simulink subsystem "PvtSubSys_VSM_ACC_DHT"  (R2020b)
settings: Solver=VariableStepAuto  StartTime=0.0  StopTime=10.0  RelTol=1e-3
values from neighbouring files (symbols this model uses):
  P_VSM_ACC_AutoGoSW = 1.0    [ACC.sldd]
  P_VSM_ACC_BOMEntry_ACCDecReqValue = -0.5    [ACC.sldd]
  P_VSM_ACC_BOMEntry_AxvRefMs2 = -0.5    [ACC.sldd]
  P_VSM_ACC_BOMExit_ACCDecReqValue = -0.3    [ACC.sldd]
  P_VSM_ACC_BrakeOnlyNum = 500.0    [ACC.sldd]
  P_VSM_ACC_RadarOffset = 0.5    [ACC.sldd]
  P_VSM_ACC_StandActiveNumACCMode = 1500.0    [ACC.sldd]
  P_VSM_ACC_StandActiveNumHWAMode = 1500.0    [ACC.sldd]
  P_VSM_ACCExit_AccOverride = 900.0    [ACC.sldd]
  P_VSM_ACCExit_StandWaitTime = 180.0    [ACC.sldd]
  P_VSM_TJA_ActiveWaitNum = 3000.0    [ACC.sldd]
undefined symbols (not defined in the file or in its folder): ACC_STATE, HWAError_Error, HWAError_ErrorBlindness, HWAError_ErrorFast, HWAError_Inhibit, TJA_STATE
libraries: simulink x130, TrueDurationTime x16
(part 2 of 2)

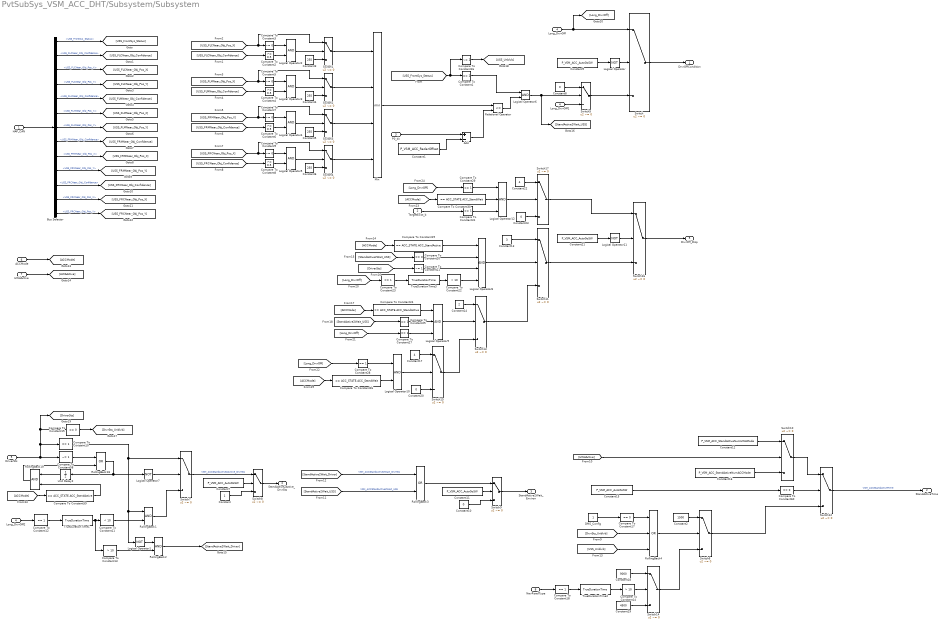
== system PvtSubSys_VSM_ACC_DHT/Subsystem/Subsystem ==
  HAP_CAN : Inport  OutDataTypeStr=Bus: HAP_CAN
  TargetExist_b : Inport  Port=2
  P0_dx : Inport  Port=3
  Long_DrvrOff : Inport  Port=4
  DriverSts : Inport  Port=5
  ACCMode : Inport  Port=6
  HWAActive : Inport  Port=7
  NavRoadType : Inport  Port=8
  Add : Sum  Inputs=+-
  Bus Selector : BusSelector  OutputSignals=USS_FrontSys_Status,USS_FLCNear_Obj_Confidence,USS_FLCNear_Obj_Pos_X,USS_FLCNear_Obj_Pos_Y,USS_FLMNear_Obj_Confidence,USS_FLMNear_Obj_Pos_X,USS_FLMNear_Obj_Pos_Y,USS_FRMNear_Obj_Confidence,USS_FRMNear_Obj_Pos_X,USS_FRMNear_Obj_Pos_Y,USS_FRCNear_Obj_Confidence,USS_FRCNear_Obj_Pos_X,USS_FRCNear_Obj_Pos_Y
  Compare To Constant1 : simulink/Logic and Bit Operations/Compare To Constant  relop===  const=2  OutDataTypeStr=boolean
  Compare To Constant16 : simulink/Logic and Bit Operations/Compare To Constant  relop=~=  const=2  OutDataTypeStr=boolean
  Compare To Constant{2,4,6,8} (4 alike) : simulink/Logic and Bit Operations/Compare To Constant  relop=>=  const=0.5  OutDataTypeStr=boolean
  Compare To Constant{15,17,20,60} (4 alike) : simulink/Logic and Bit Operations/Compare To Constant  relop===  const=0  OutDataTypeStr=boolean
  Compare To Constant21 : simulink/Logic and Bit Operations/Compare To Constant  relop=~=  const=1  OutDataTypeStr=boolean
  Compare To Constant{10,12,18,23,25,27..29,31} (9 alike) : simulink/Logic and Bit Operations/Compare To Constant  relop===  const=1  OutDataTypeStr=boolean
  Compare To Constant{3,5,7,9} (4 alike) : simulink/Logic and Bit Operations/Compare To Constant  relop=~=  const=0  OutDataTypeStr=boolean
  Compare To Constant11 : simulink/Logic and Bit Operations/Compare To Constant  relop=<  const=10  OutDataTypeStr=boolean
  Compare To Constant13 : simulink/Logic and Bit Operations/Compare To Constant  relop=>  const=10  OutDataTypeStr=boolean
  Compare To Constant14 : simulink/Logic and Bit Operations/Compare To Constant  relop=>  const=10  OutDataTypeStr=boolean
  Compare To Constant19 : simulink/Logic and Bit Operations/Compare To Constant  relop===  const=ACC_STATE.ACC_StandActive  OutDataTypeStr=boolean
  Compare To Constant22 : simulink/Logic and Bit Operations/Compare To Constant  relop=<  const=10  OutDataTypeStr=boolean
  Compare To Constant24 : simulink/Logic and Bit Operations/Compare To Constant  relop===  const=ACC_STATE.ACC_StandActive  OutDataTypeStr=boolean
  Compare To Constant26 : simulink/Logic and Bit Operations/Compare To Constant  relop===  const=ACC_STATE.ACC_StandWait  OutDataTypeStr=boolean
  Compare To Constant30 : simulink/Logic and Bit Operations/Compare To Constant  relop===  const=ACC_STATE.ACC_StandWait  OutDataTypeStr=boolean
  Compare To Constant58 : simulink/Logic and Bit Operations/Compare To Constant  relop=~=  const=1  OutDataTypeStr=boolean
  Compare To Constant59 : simulink/Logic and Bit Operations/Compare To Constant  relop===  const=ACC_STATE.ACC_StandActive  OutDataTypeStr=boolean
  Constant : Constant  OutDataTypeStr=boolean
  Constant1 : Constant  Value=P_VSM_ACC_RadarOffset
  Constant10 : Constant  Value=0  OutDataTypeStr=boolean
  Constant{7,9,11,15,21} (5 alike) : Constant  Value=P_VSM_ACC_AutoGoSW  VectorParams1D=off  SampleTime=-1
  Constant12 : Constant  Value=P_VSM_ACC_StandActiveNumHWAMode  VectorParams1D=off  SampleTime=-1
  Constant13 : Constant  Value=3  OutDataTypeStr=uint8
  Constant14 : Constant  Value=2  OutDataTypeStr=uint8
  Constant16 : Constant  Value=P_VSM_ACC_StandActiveNumACCMode  VectorParams1D=off  SampleTime=-1
  Constant17 : Constant  Value=4  OutDataTypeStr=uint8
  Constant18 : Constant  Value=9000  VectorParams1D=off  OutDataTypeStr=uint16  SampleTime=-1
  Constant19 : Constant  Value=4500  VectorParams1D=off  OutDataTypeStr=uint16  SampleTime=-1
  Constant2 : Constant  Value=1500  VectorParams1D=off  OutDataTypeStr=uint16  SampleTime=-1
  Constant20 : Constant  Value=0  OutDataTypeStr=uint8
  Constant22 : Constant  Value=4  OutDataTypeStr=uint8
  Constant23 : Constant  Value=0  OutDataTypeStr=uint8
  Constant{3..6} (4 alike) : Constant  Value=255  OutDataTypeStr=single
  Constant8 : Constant  Value=0  OutDataTypeStr=boolean
  DMS_Config : Constant  OutDataTypeStr=boolean
  Logical Operator{,1,7,11} (4 alike) : Logic  Operator=NOT  Inputs=1  AllPortsSameDT=off  OutDataTypeStr=boolean
  Logical Operator{2..6,10} (6 alike) : Logic  AllPortsSameDT=off  OutDataTypeStr=boolean
  Logical Operator12 : Logic  Inputs=3  AllPortsSameDT=off  OutDataTypeStr=boolean
  Logical Operator8 : Logic  Inputs=4  AllPortsSameDT=off  OutDataTypeStr=boolean
  Logical Operator9 : Logic  Inputs=3  AllPortsSameDT=off  OutDataTypeStr=boolean
  Long_DrvrOff1 : InportShadow  Port=4
  Long_DrvrOff2 : InportShadow  Port=4
  Min : MinMax  Inputs=4
  Relational Operator : RelationalOperator  Operator=<=  OutDataTypeStr=boolean  RndMeth=Simplest
  RollingBack1 : Logic  AllPortsSameDT=off  OutDataTypeStr=boolean
  RollingBack18 : Logic  Operator=OR  AllPortsSameDT=off  OutDataTypeStr=boolean
  RollingBack19 : Logic  AllPortsSameDT=off  OutDataTypeStr=boolean
  RollingBack2 : Logic  AllPortsSameDT=off  OutDataTypeStr=boolean
  RollingBack3 : Logic  Operator=OR  AllPortsSameDT=off  OutDataTypeStr=boolean
  RollingBack4 : Logic  Operator=OR  Inputs=3  AllPortsSameDT=off  OutDataTypeStr=boolean
  Switch{,1..17} (18 alike) : Switch  Criteria=u2 ~= 0
  TrueDurationTime1 : TrueDurationTime/TrueDurationTime  TCycle=0.02
  TrueDurationTime2 : TrueDurationTime/TrueDurationTime  TCycle=0.02
  TrueDurationTime3 : TrueDurationTime/TrueDurationTime  TCycle=0.02
  Unit Delay2 : UnitDelay  SampleTime=-1  HasFrameUpgradeWarning=on
  DrvrOffCondition : Outport
  StandActiveTime : Outport  Port=2
  StandActive2Wait_Environ : Outport  Port=3
  StandActive2Active_DrvrSts : Outport  Port=4
  DrvrOff_Disp : Outport  Port=5
  wires:
  Switch/1 -> DrvrOffCondition/1
  Long_DrvrOff/1 -> [Long_DrvrOff], Switch/1
  Constant9/1 -> Logical Operator/1
  Logical Operator/1 -> Switch/2
  [USS_FrontSys_Status] -> Compare To Constant16/1, Compare To Constant1/1
  [USS_FLCNear_Obj_Confidence] -> Compare To Constant2/1
  Logical Operator2/1 -> Switch1/2
  Compare To Constant2/1 -> Logical Operator2/2
  [USS_FLCNear_Obj_Pos_X] -> Switch1/1, Compare To Constant3/1
  Compare To Constant3/1 -> Logical Operator2/1
  Constant3/1 -> Switch1/3
  Constant4/1 -> Switch2/3
  Compare To Constant5/1 -> Logical Operator3/1
  [USS_FLMNear_Obj_Pos_X] -> Compare To Constant5/1, Switch2/1
  Compare To Constant4/1 -> Logical Operator3/2
  Logical Operator3/1 -> Switch2/2
  [USS_FLMNear_Obj_Confidence] -> Compare To Constant4/1
  [USS_FRMNear_Obj_Confidence] -> Compare To Constant6/1
  Logical Operator4/1 -> Switch3/2
  Compare To Constant6/1 -> Logical Operator4/2
  [USS_FRMNear_Obj_Pos_X] -> Switch3/1, Compare To Constant7/1
  Compare To Constant7/1 -> Logical Operator4/1
  Constant5/1 -> Switch3/3
  Constant6/1 -> Switch4/3
  Compare To Constant9/1 -> Logical Operator5/1
  [USS_FRCNear_Obj_Pos_X] -> Compare To Constant9/1, Switch4/1
  Compare To Constant8/1 -> Logical Operator5/2
  Logical Operator5/1 -> Switch4/2
  [USS_FRCNear_Obj_Confidence] -> Compare To Constant8/1
  Switch2/1 -> Min/2
  Switch1/1 -> Min/1
  Switch3/1 -> Min/3
  Switch4/1 -> Min/4
  Min/1 -> Relational Operator/1
  P0_dx/1 -> Add/1
  Add/1 -> Relational Operator/2
  Constant1/1 -> Add/2
  Compare To Constant1/1 -> Logical Operator6/1
  Relational Operator/1 -> Logical Operator6/2
  Logical Operator6/1 -> [StandActive2Wait_USS], Switch5/2
  Constant8/1 -> Switch5/1
  Long_DrvrOff1/1 -> Switch5/3
  Switch5/1 -> Switch/3
  HAP_CAN/1 -> Bus Selector/1
  Bus Selector/3 -> [USS_FLCNear_Obj_Pos_X]  "<USS_FLCNear_Obj_Pos_X>"
  Bus Selector/2 -> [USS_FLCNear_Obj_Confidence]  "<USS_FLCNear_Obj_Confidence>"
  Bus Selector/4 -> [USS_FLCNear_Obj_Pos_Y]  "<USS_FLCNear_Obj_Pos_Y>"
  Bus Selector/1 -> [USS_FrontSys_Status]  "<USS_FrontSys_Status>"
  Bus Selector/7 -> [USS_FLMNear_Obj_Pos_Y]  "<USS_FLMNear_Obj_Pos_Y>"
  Bus Selector/6 -> [USS_FLMNear_Obj_Pos_X]  "<USS_FLMNear_Obj_Pos_X>"
  Bus Selector/5 -> [USS_FLMNear_Obj_Confidence]  "<USS_FLMNear_Obj_Confidence>"
  Bus Selector/10 -> [USS_FRMNear_Obj_Pos_Y]  "<USS_FRMNear_Obj_Pos_Y>"
  Bus Selector/9 -> [USS_FRMNear_Obj_Pos_X]  "<USS_FRMNear_Obj_Pos_X>"
  Bus Selector/8 -> [USS_FRMNear_Obj_Confidence]  "<USS_FRMNear_Obj_Confidence>"
  Bus Selector/11 -> [USS_FRCNear_Obj_Confidence]  "<USS_FRCNear_Obj_Confidence>"
  Bus Selector/12 -> [USS_FRCNear_Obj_Pos_X]  "<USS_FRCNear_Obj_Pos_X>"
  Bus Selector/13 -> [USS_FRCNear_Obj_Pos_Y]  "<USS_FRCNear_Obj_Pos_Y>"
  Logical Operator7/1 -> Switch7/2
  Compare To Constant58/1 -> RollingBack18/1
  Switch12/1 -> StandActiveTime/1  "VSM_ACCStandActiveTime"
  [ACCMode] -> Compare To Constant59/1
  RollingBack18/1 -> Unit Delay2/1, Logical Operator7/1
  Compare To Constant59/1 -> RollingBack19/2
  Unit Delay2/1 -> RollingBack19/1
  RollingBack19/1 -> RollingBack18/2
  ACCMode/1 -> [ACCMode]
  HWAActive/1 -> [HWAActive]
  DriverSts/1 -> Compare To Constant10/1, Compare To Constant15/1, [DriverSts], Compare To Constant58/1
  Compare To Constant10/1 -> Logical Operator1/1, RollingBack1/1, Switch7/1
  RollingBack1/1 -> Switch7/3
  TrueDurationTime1/1 -> Compare To Constant13/1, Compare To Constant11/1
  Compare To Constant11/1 -> RollingBack1/2
  Long_DrvrOff2/1 -> Compare To Constant12/1
  Compare To Constant12/1 -> TrueDurationTime1/1
  Logical Operator1/1 -> RollingBack2/1
  Compare To Constant13/1 -> RollingBack2/2
  RollingBack2/1 -> [StandActive2Wait_Driver]
  [StandActive2Wait_Driver] -> RollingBack3/1  "VSM_ACCStandActive2Wait_DrvrSts"
  [StandActive2Wait_USS] -> RollingBack3/2  "VSM_ACCStandActive2Wait_USS"
  RollingBack3/1 -> Switch9/1
  Switch7/1 -> Switch8/1  "VSM_ACCStandActive2Active_DrvrSts"
  Switch8/1 -> StandActive2Active_DrvrSts/1
  Constant7/1 -> Switch8/2
  Constant/1 -> Switch8/3
  Constant10/1 -> Switch9/3
  Constant11/1 -> Switch9/2
  Switch9/1 -> StandActive2Wait_Environ/1
  [HWAActive] -> Switch10/2
  Constant12/1 -> Switch10/1
  Switch6/1 -> Switch12/3
  Switch10/1 -> Switch12/1
  Constant15/1 -> Compare To Constant60/1
  Compare To Constant60/1 -> Switch12/2
  Constant16/1 -> Switch10/3
  Compare To Constant15/1 -> [DrvrSts_Unblvb]
  Compare To Constant16/1 -> [USS_Unblvb]
  DMS_Config/1 -> Compare To Constant17/1
  Compare To Constant17/1 -> RollingBack4/1
  [DrvrSts_Unblvb] -> RollingBack4/2
  [USS_Unblvb] -> RollingBack4/3
  RollingBack4/1 -> Switch6/2
  Constant2/1 -> Switch6/1
  Switch14/1 -> Switch6/3
  NavRoadType/1 -> Compare To Constant18/1
  Compare To Constant18/1 -> TrueDurationTime2/1
  Constant18/1 -> Switch14/1
  Constant19/1 -> Switch14/3
  TrueDurationTime2/1 -> Compare To Constant14/1
  Compare To Constant14/1 -> Switch14/2
  [ACCMode] -> Compare To Constant19/1
  Logical Operator8/1 -> Switch11/2
  Compare To Constant19/1 -> Logical Operator8/1
  [StandActive2Wait_USS] -> Compare To Constant20/1
  Compare To Constant20/1 -> Logical Operator8/2
  Compare To Constant21/1 -> Logical Operator8/3
  [DriverSts] -> Compare To Constant21/1
  Compare To Constant23/1 -> TrueDurationTime3/1
  TrueDurationTime3/1 -> Compare To Constant22/1
  [Long_DrvrOff] -> Compare To Constant23/1
  Compare To Constant22/1 -> Logical Operator8/4
  Constant13/1 -> Switch11/1
  Switch13/1 -> Switch11/3
  Logical Operator9/1 -> Switch13/2
  [ACCMode] -> Compare To Constant24/1
  Compare To Constant24/1 -> Logical Operator9/1
  [StandActive2Wait_USS] -> Compare To Constant25/1
  Compare To Constant25/1 -> Logical Operator9/2
  Constant14/1 -> Switch13/1
  [ACCMode] -> Compare To Constant26/1
  Switch15/1 -> Switch13/3
  Logical Operator10/1 -> Switch15/2
  Compare To Constant26/1 -> Logical Operator10/2
  [Long_DrvrOff] -> Compare To Constant27/1
  Compare To Constant27/1 -> Logical Operator9/3
  Compare To Constant28/1 -> Logical Operator10/1
  [Long_DrvrOff] -> Compare To Constant28/1
  Constant17/1 -> Switch15/1
  Constant20/1 -> Switch15/3
  Logical Operator11/1 -> Switch16/2
  Constant21/1 -> Logical Operator11/1
  Switch11/1 -> Switch16/3
  Constant23/1 -> Switch17/3
  Constant22/1 -> Switch17/1
  [Long_DrvrOff] -> Compare To Constant29/1
  Compare To Constant29/1 -> Logical Operator12/1
  Compare To Constant30/1 -> Logical Operator12/2
  Logical Operator12/1 -> Switch17/2
  [ACCMode] -> Compare To Constant30/1
  Switch17/1 -> Switch16/1
  TargetExist_b/1 -> Compare To Constant31/1
  Compare To Constant31/1 -> Logical Operator12/3
  Switch16/1 -> DrvrOff_Disp/1

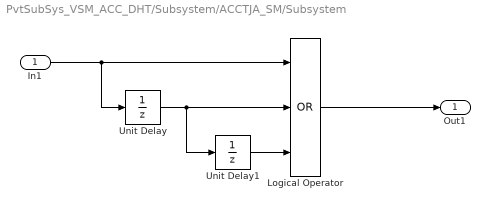
== system PvtSubSys_VSM_ACC_DHT/Subsystem/ACCTJA_SM/Subsystem ==
  In1 : Inport
  Logical Operator : Logic  Operator=OR  Inputs=3  AllPortsSameDT=off  OutDataTypeStr=boolean
  Unit Delay : UnitDelay  SampleTime=-1  HasFrameUpgradeWarning=on
  Unit Delay1 : UnitDelay  SampleTime=-1  HasFrameUpgradeWarning=on
  Out1 : Outport
  wires:
  In1/1 -> Logical Operator/1, Unit Delay/1
  Unit Delay/1 -> Logical Operator/2, Unit Delay1/1
  Logical Operator/1 -> Out1/1
  Unit Delay1/1 -> Logical Operator/3

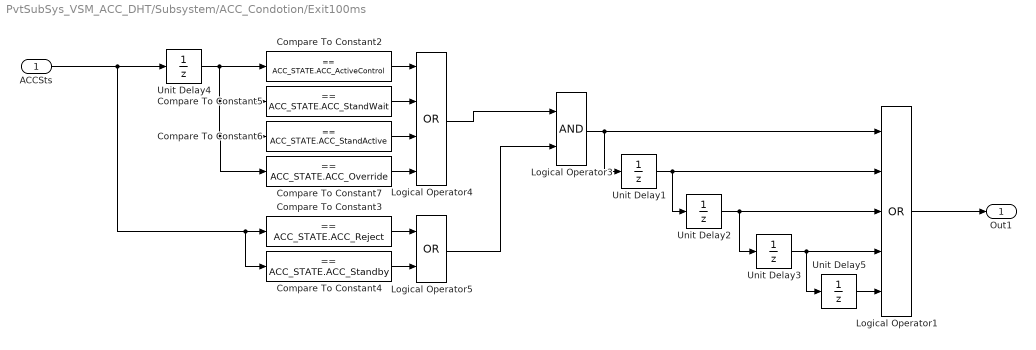
== system PvtSubSys_VSM_ACC_DHT/Subsystem/ACC_Condotion/Exit100ms ==
  ACCSts : Inport
  Compare To Constant2 : simulink/Logic and Bit Operations/Compare To Constant  relop===  const=ACC_STATE.ACC_ActiveControl  OutDataTypeStr=boolean
  Compare To Constant3 : simulink/Logic and Bit Operations/Compare To Constant  relop===  const=ACC_STATE.ACC_Reject  OutDataTypeStr=boolean
  Compare To Constant4 : simulink/Logic and Bit Operations/Compare To Constant  relop===  const=ACC_STATE.ACC_Standby  OutDataTypeStr=boolean
  Compare To Constant5 : simulink/Logic and Bit Operations/Compare To Constant  relop===  const=ACC_STATE.ACC_StandWait  OutDataTypeStr=boolean
  Compare To Constant6 : simulink/Logic and Bit Operations/Compare To Constant  relop===  const=ACC_STATE.ACC_StandActive  OutDataTypeStr=boolean
  Compare To Constant7 : simulink/Logic and Bit Operations/Compare To Constant  relop===  const=ACC_STATE.ACC_Override  OutDataTypeStr=boolean
  Logical Operator1 : Logic  Operator=OR  Inputs=5  AllPortsSameDT=off  OutDataTypeStr=boolean
  Logical Operator3 : Logic  AllPortsSameDT=off  OutDataTypeStr=boolean
  Logical Operator4 : Logic  Operator=OR  Inputs=4  AllPortsSameDT=off  OutDataTypeStr=boolean
  Logical Operator5 : Logic  Operator=OR  AllPortsSameDT=off  OutDataTypeStr=boolean
  Unit Delay{1..3,5} (4 alike) : UnitDelay  SampleTime=-1  HasFrameUpgradeWarning=on
  Unit Delay4 : UnitDelay  InitialCondition=ACC_STATE.ACC_Off  SampleTime=-1  HasFrameUpgradeWarning=on
  Out1 : Outport
  wires:
  Unit Delay5/1 -> Logical Operator1/5
  Unit Delay3/1 -> Logical Operator1/4, Unit Delay5/1
  Unit Delay2/1 -> Logical Operator1/3, Unit Delay3/1
  Unit Delay1/1 -> Logical Operator1/2, Unit Delay2/1
  Logical Operator3/1 -> Unit Delay1/1, Logical Operator1/1
  Compare To Constant7/1 -> Logical Operator4/4
  Compare To Constant6/1 -> Logical Operator4/3
  Compare To Constant5/1 -> Logical Operator4/2
  Compare To Constant2/1 -> Logical Operator4/1
  Compare To Constant3/1 -> Logical Operator5/1
  Compare To Constant4/1 -> Logical Operator5/2
  ACCSts/1 -> Compare To Constant4/1, Compare To Constant3/1, Unit Delay4/1
  Unit Delay4/1 -> Compare To Constant5/1, Compare To Constant6/1, Compare To Constant7/1, Compare To Constant2/1
  Logical Operator4/1 -> Logical Operator3/1
  Logical Operator1/1 -> Out1/1
  Logical Operator5/1 -> Logical Operator3/2

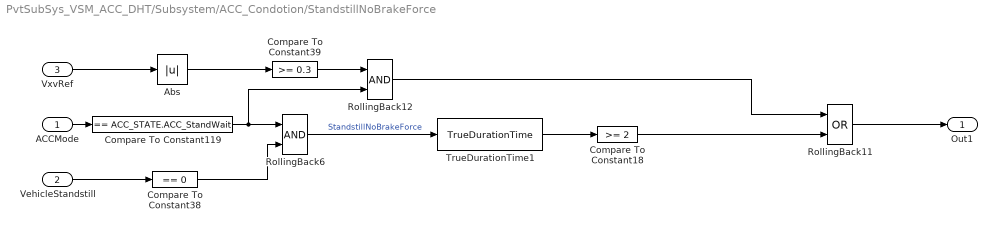
== system PvtSubSys_VSM_ACC_DHT/Subsystem/ACC_Condotion/StandstillNoBrakeForce ==
  ACCMode : Inport
  VehicleStandstill : Inport  Port=2
  VxvRef : Inport  Port=3
  Abs : Abs
  Compare To Constant119 : simulink/Logic and Bit Operations/Compare To Constant  relop===  const=ACC_STATE.ACC_StandWait  OutDataTypeStr=boolean
  Compare To Constant18 : simulink/Logic and Bit Operations/Compare To Constant  relop=>=  const=2  OutDataTypeStr=boolean
  Compare To Constant38 : simulink/Logic and Bit Operations/Compare To Constant  relop===  const=0  OutDataTypeStr=boolean
  Compare To Constant39 : simulink/Logic and Bit Operations/Compare To Constant  relop=>=  const=0.3  OutDataTypeStr=boolean
  RollingBack11 : Logic  Operator=OR  AllPortsSameDT=off  OutDataTypeStr=boolean
  RollingBack12 : Logic  AllPortsSameDT=off  OutDataTypeStr=boolean
  RollingBack6 : Logic  AllPortsSameDT=off  OutDataTypeStr=boolean
  TrueDurationTime1 : TrueDurationTime/TrueDurationTime  TCycle=0.02
  Out1 : Outport
  wires:
  Abs/1 -> Compare To Constant39/1
  Compare To Constant119/1 -> RollingBack6/1, RollingBack12/2
  RollingBack6/1 -> TrueDurationTime1/1  "StandstillNoBrakeForce"
  TrueDurationTime1/1 -> Compare To Constant18/1
  Compare To Constant38/1 -> RollingBack6/2
  VehicleStandstill/1 -> Compare To Constant38/1
  Compare To Constant39/1 -> RollingBack12/1
  RollingBack12/1 -> RollingBack11/1
  RollingBack11/1 -> Out1/1
  VxvRef/1 -> Abs/1
  Compare To Constant18/1 -> RollingBack11/2
  ACCMode/1 -> Compare To Constant119/1

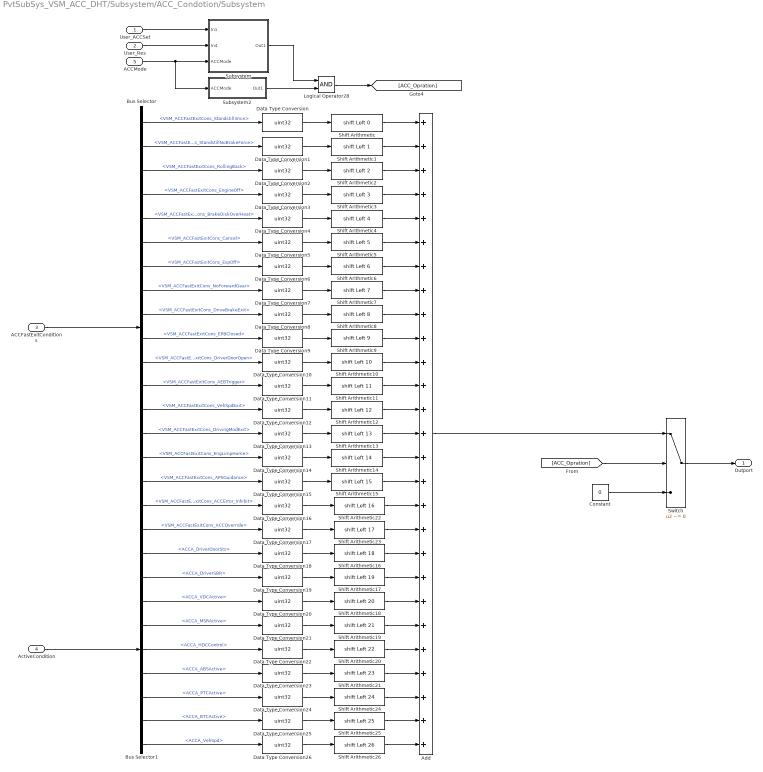
== system PvtSubSys_VSM_ACC_DHT/Subsystem/ACC_Condotion/Subsystem ==
  User_ACCSet : Inport
  User_Res : Inport  Port=2
  ACCFastExitConditions : Inport  Port=3
  ActiveCondition : Inport  Port=4
  ACCMode : Inport  Port=5
  Add : Sum  Inputs=+++++++++++++++++++++++++++
  Bus Selector : BusSelector  OutputSignals=VSM_ACCFastExitCons_Standstill3min,VSM_ACCFastExitCons_StandstillNoBrakeForce,VSM_ACCFastExitCons_RollingBack,VSM_ACCFastExitCons_EngineOff,VSM_ACCFastExitCons_BrakeDiskOverHeat,VSM_ACCFastExitCons_Cancel,VSM_ACCFastExitCons_EspOff,VSM_ACCFastExitCons_NoForwardGear,VSM_ACCFastExitCons_DriveBrakeExit,VSM_ACCFastExitCons_EPBClosed,VSM_ACCFastExitCons_DriverDoorOpen,VSM_ACCFastExitCons_AEBTrigger,VSM_ACCFastExitCons_VehSpdExit,VSM_ACCFastExitCons_DrivingModExit,VSM_ACCFastExitCons_EngLimpHome,VSM_ACCFastExitCons_APSGuidance,VSM_ACCFastExitCons_ACCError_Inhibit,VSM_ACCFastExitCons_ACCOverride
  Bus Selector1 : BusSelector  OutputSignals=ACCA_DriverDoorSts,ACCA_DriverSBR,ACCA_VDCActive,ACCA_MSRActive,ACCA_HDCControl,ACCA_ABSActive,ACCA_PTCActive,ACCA_BTCActive,ACCA_VehSpd
  Constant : Constant  Value=0  OutDataTypeStr=uint32
  Data Type Conversion{,1..26} (27 alike) : DataTypeConversion  OutDataTypeStr=uint32
  Logical Operator28 : Logic  AllPortsSameDT=off  OutDataTypeStr=boolean
  Shift Arithmetic : ArithShift  BitShiftDirection=Left
  Shift Arithmetic1 : ArithShift  BitShiftNumber=1  BitShiftDirection=Left
  Shift Arithmetic10 : ArithShift  BitShiftNumber=10  BitShiftDirection=Left
  Shift Arithmetic11 : ArithShift  BitShiftNumber=11  BitShiftDirection=Left
  Shift Arithmetic12 : ArithShift  BitShiftNumber=12  BitShiftDirection=Left
  Shift Arithmetic13 : ArithShift  BitShiftNumber=13  BitShiftDirection=Left
  Shift Arithmetic14 : ArithShift  BitShiftNumber=14  BitShiftDirection=Left
  Shift Arithmetic15 : ArithShift  BitShiftNumber=15  BitShiftDirection=Left
  Shift Arithmetic16 : ArithShift  BitShiftNumber=18  BitShiftDirection=Left
  Shift Arithmetic17 : ArithShift  BitShiftNumber=19  BitShiftDirection=Left
  Shift Arithmetic18 : ArithShift  BitShiftNumber=20  BitShiftDirection=Left
  Shift Arithmetic19 : ArithShift  BitShiftNumber=21  BitShiftDirection=Left
  Shift Arithmetic2 : ArithShift  BitShiftNumber=2  BitShiftDirection=Left
  Shift Arithmetic20 : ArithShift  BitShiftNumber=22  BitShiftDirection=Left
  Shift Arithmetic21 : ArithShift  BitShiftNumber=23  BitShiftDirection=Left
  Shift Arithmetic22 : ArithShift  BitShiftNumber=16  BitShiftDirection=Left
  Shift Arithmetic23 : ArithShift  BitShiftNumber=17  BitShiftDirection=Left
  Shift Arithmetic24 : ArithShift  BitShiftNumber=24  BitShiftDirection=Left
  Shift Arithmetic25 : ArithShift  BitShiftNumber=25  BitShiftDirection=Left
  Shift Arithmetic26 : ArithShift  BitShiftNumber=26  BitShiftDirection=Left
  Shift Arithmetic3 : ArithShift  BitShiftNumber=3  BitShiftDirection=Left
  Shift Arithmetic4 : ArithShift  BitShiftNumber=4  BitShiftDirection=Left
  Shift Arithmetic5 : ArithShift  BitShiftNumber=5  BitShiftDirection=Left
  Shift Arithmetic6 : ArithShift  BitShiftNumber=6  BitShiftDirection=Left
  Shift Arithmetic7 : ArithShift  BitShiftNumber=7  BitShiftDirection=Left
  Shift Arithmetic8 : ArithShift  BitShiftNumber=8  BitShiftDirection=Left
  Shift Arithmetic9 : ArithShift  BitShiftNumber=9  BitShiftDirection=Left
  Subsystem : Subsystem
  Subsystem2 : Subsystem
  Switch : Switch  Criteria=u2 ~= 0
  Outport : Outport
  wires:
  Switch/1 -> Outport/1
  [ACC_Opration] -> Switch/2
  Logical Operator28/1 -> [ACC_Opration]
  Subsystem2/1(Out1) -> Logical Operator28/2
  Subsystem/1(Out1) -> Logical Operator28/1
  User_Res/1 -> Subsystem/2(In4)
  ACCMode/1 -> Subsystem/3(ACCMode), Subsystem2/1(ACCMode)
  User_ACCSet/1 -> Subsystem/1(In1)
  Constant/1 -> Switch/3
  Add/1 -> Switch/1
  Shift Arithmetic15/1 -> Add/16
  Shift Arithmetic14/1 -> Add/15
  Shift Arithmetic13/1 -> Add/14
  Shift Arithmetic12/1 -> Add/13
  Shift Arithmetic11/1 -> Add/12
  Shift Arithmetic10/1 -> Add/11
  Shift Arithmetic9/1 -> Add/10
  Shift Arithmetic8/1 -> Add/9
  Shift Arithmetic7/1 -> Add/8
  Shift Arithmetic6/1 -> Add/7
  Shift Arithmetic5/1 -> Add/6
  Shift Arithmetic4/1 -> Add/5
  Shift Arithmetic3/1 -> Add/4
  Shift Arithmetic2/1 -> Add/3
  Shift Arithmetic1/1 -> Add/2
  Shift Arithmetic/1 -> Add/1
  Shift Arithmetic26/1 -> Add/27
  Shift Arithmetic25/1 -> Add/26
  Shift Arithmetic24/1 -> Add/25
  Shift Arithmetic21/1 -> Add/24
  Shift Arithmetic20/1 -> Add/23
  Shift Arithmetic19/1 -> Add/22
  Shift Arithmetic18/1 -> Add/21
  Shift Arithmetic17/1 -> Add/20
  Shift Arithmetic16/1 -> Add/19
  Shift Arithmetic23/1 -> Add/18
  Shift Arithmetic22/1 -> Add/17
  Data Type Conversion26/1 -> Shift Arithmetic26/1
  Data Type Conversion25/1 -> Shift Arithmetic25/1
  Data Type Conversion24/1 -> Shift Arithmetic24/1
  Data Type Conversion23/1 -> Shift Arithmetic21/1
  Data Type Conversion22/1 -> Shift Arithmetic20/1
  Data Type Conversion21/1 -> Shift Arithmetic19/1
  Data Type Conversion20/1 -> Shift Arithmetic18/1
  Data Type Conversion19/1 -> Shift Arithmetic17/1
  Data Type Conversion18/1 -> Shift Arithmetic16/1
  Data Type Conversion17/1 -> Shift Arithmetic23/1
  Data Type Conversion16/1 -> Shift Arithmetic22/1
  Data Type Conversion15/1 -> Shift Arithmetic15/1
  Data Type Conversion14/1 -> Shift Arithmetic14/1
  Data Type Conversion13/1 -> Shift Arithmetic13/1
  Data Type Conversion12/1 -> Shift Arithmetic12/1
  Data Type Conversion11/1 -> Shift Arithmetic11/1
  Data Type Conversion10/1 -> Shift Arithmetic10/1
  Data Type Conversion9/1 -> Shift Arithmetic9/1
  Data Type Conversion8/1 -> Shift Arithmetic8/1
  Data Type Conversion7/1 -> Shift Arithmetic7/1
  Data Type Conversion6/1 -> Shift Arithmetic6/1
  Data Type Conversion5/1 -> Shift Arithmetic5/1
  Data Type Conversion4/1 -> Shift Arithmetic4/1
  Data Type Conversion3/1 -> Shift Arithmetic3/1
  Data Type Conversion2/1 -> Shift Arithmetic2/1
  Data Type Conversion1/1 -> Shift Arithmetic1/1
  Data Type Conversion/1 -> Shift Arithmetic/1
  Bus Selector1/9 -> Data Type Conversion26/1  "<ACCA_VehSpd>"
  Bus Selector1/8 -> Data Type Conversion25/1  "<ACCA_BTCActive>"
  Bus Selector1/7 -> Data Type Conversion24/1  "<ACCA_PTCActive>"
  Bus Selector1/6 -> Data Type Conversion23/1  "<ACCA_ABSActive>"
  Bus Selector1/5 -> Data Type Conversion22/1  "<ACCA_HDCControl>"
  Bus Selector1/4 -> Data Type Conversion21/1  "<ACCA_MSRActive>"
  Bus Selector1/3 -> Data Type Conversion20/1  "<ACCA_VDCActive>"
  Bus Selector1/1 -> Data Type Conversion18/1  "<ACCA_DriverDoorSts>"
  Bus Selector1/2 -> Data Type Conversion19/1  "<ACCA_DriverSBR>"
  Bus Selector/18 -> Data Type Conversion17/1  "<VSM_ACCFastExitCons_ACCOverride>"
  Bus Selector/17 -> Data Type Conversion16/1  "<VSM_ACCFastExitCons_ACCError_Inhibit>"
  Bus Selector/16 -> Data Type Conversion15/1  "<VSM_ACCFastExitCons_APSGuidance>"
  Bus Selector/15 -> Data Type Conversion14/1  "<VSM_ACCFastExitCons_EngLimpHome>"
  Bus Selector/14 -> Data Type Conversion13/1  "<VSM_ACCFastExitCons_DrivingModExit>"
  Bus Selector/13 -> Data Type Conversion12/1  "<VSM_ACCFastExitCons_VehSpdExit>"
  Bus Selector/12 -> Data Type Conversion11/1  "<VSM_ACCFastExitCons_AEBTrigger>"
  Bus Selector/11 -> Data Type Conversion10/1  "<VSM_ACCFastExitCons_DriverDoorOpen>"
  Bus Selector/10 -> Data Type Conversion9/1  "<VSM_ACCFastExitCons_EPBClosed>"
  Bus Selector/9 -> Data Type Conversion8/1  "<VSM_ACCFastExitCons_DriveBrakeExit>"
  Bus Selector/8 -> Data Type Conversion7/1  "<VSM_ACCFastExitCons_NoForwardGear>"
  Bus Selector/7 -> Data Type Conversion6/1  "<VSM_ACCFastExitCons_EspOff>"
  Bus Selector/6 -> Data Type Conversion5/1  "<VSM_ACCFastExitCons_Cancel>"
  Bus Selector/5 -> Data Type Conversion4/1  "<VSM_ACCFastExitCons_BrakeDiskOverHeat>"
  Bus Selector/4 -> Data Type Conversion3/1  "<VSM_ACCFastExitCons_EngineOff>"
  Bus Selector/3 -> Data Type Conversion2/1  "<VSM_ACCFastExitCons_RollingBack>"
  Bus Selector/2 -> Data Type Conversion1/1  "<VSM_ACCFastExitCons_StandstillNoBrakeForce>"
  Bus Selector/1 -> Data Type Conversion/1  "<VSM_ACCFastExitCons_Standstill3min>"
  ActiveCondition/1 -> Bus Selector1/1
  ACCFastExitConditions/1 -> Bus Selector/1

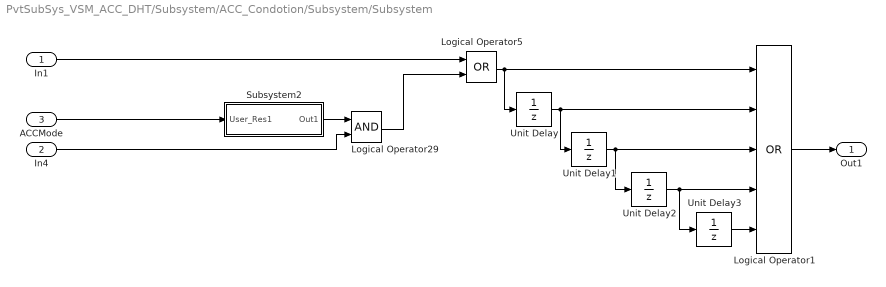
== system PvtSubSys_VSM_ACC_DHT/Subsystem/ACC_Condotion/Subsystem/Subsystem ==
  In1 : Inport
  In4 : Inport  Port=2
  ACCMode : Inport  Port=3
  Logical Operator1 : Logic  Operator=OR  Inputs=5  AllPortsSameDT=off  OutDataTypeStr=boolean
  Logical Operator29 : Logic  AllPortsSameDT=off  OutDataTypeStr=boolean
  Logical Operator5 : Logic  Operator=OR  AllPortsSameDT=off  OutDataTypeStr=boolean
  Subsystem2 : Subsystem
  Unit Delay{,1..3} (4 alike) : UnitDelay  SampleTime=-1  HasFrameUpgradeWarning=on
  Out1 : Outport
  wires:
  Unit Delay3/1 -> Logical Operator1/5
  Unit Delay2/1 -> Logical Operator1/4, Unit Delay3/1
  Unit Delay1/1 -> Logical Operator1/3, Unit Delay2/1
  Logical Operator1/1 -> Out1/1
  Unit Delay/1 -> Logical Operator1/2, Unit Delay1/1
  In1/1 -> Logical Operator5/1
  Logical Operator5/1 -> Unit Delay/1, Logical Operator1/1
  In4/1 -> Logical Operator29/2
  ACCMode/1 -> Subsystem2/1(User_Res1)
  Logical Operator29/1 -> Logical Operator5/2
  Subsystem2/1(Out1) -> Logical Operator29/1

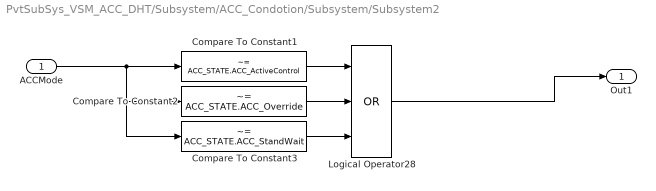
== system PvtSubSys_VSM_ACC_DHT/Subsystem/ACC_Condotion/Subsystem/Subsystem2 ==
  ACCMode : Inport
  Compare To Constant1 : simulink/Logic and Bit Operations/Compare To Constant  relop=~=  const=ACC_STATE.ACC_ActiveControl  OutDataTypeStr=boolean
  Compare To Constant2 : simulink/Logic and Bit Operations/Compare To Constant  relop=~=  const=ACC_STATE.ACC_Override  OutDataTypeStr=boolean
  Compare To Constant3 : simulink/Logic and Bit Operations/Compare To Constant  relop=~=  const=ACC_STATE.ACC_StandWait  OutDataTypeStr=boolean
  Logical Operator28 : Logic  Operator=OR  Inputs=3  AllPortsSameDT=off  OutDataTypeStr=boolean
  Out1 : Outport
  wires:
  Compare To Constant3/1 -> Logical Operator28/3
  Compare To Constant2/1 -> Logical Operator28/2
  Compare To Constant1/1 -> Logical Operator28/1
  ACCMode/1 -> Compare To Constant1/1, Compare To Constant2/1, Compare To Constant3/1
  Logical Operator28/1 -> Out1/1

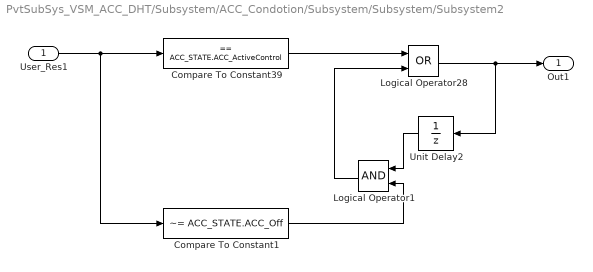
== system PvtSubSys_VSM_ACC_DHT/Subsystem/ACC_Condotion/Subsystem/Subsystem/Subsystem2 ==
  User_Res1 : Inport
  Compare To Constant1 : simulink/Logic and Bit Operations/Compare To Constant  relop=~=  const=ACC_STATE.ACC_Off  OutDataTypeStr=boolean
  Compare To Constant39 : simulink/Logic and Bit Operations/Compare To Constant  relop===  const=ACC_STATE.ACC_ActiveControl  OutDataTypeStr=boolean
  Logical Operator1 : Logic  AllPortsSameDT=off  OutDataTypeStr=boolean
  Logical Operator28 : Logic  Operator=OR  AllPortsSameDT=off  OutDataTypeStr=boolean
  Unit Delay2 : UnitDelay  SampleTime=-1  HasFrameUpgradeWarning=on
  Out1 : Outport
  wires:
  Compare To Constant1/1 -> Logical Operator1/2
  Logical Operator1/1 -> Logical Operator28/2
  User_Res1/1 -> Compare To Constant1/1, Compare To Constant39/1
  Unit Delay2/1 -> Logical Operator1/1
  Logical Operator28/1 -> Unit Delay2/1, Out1/1
  Compare To Constant39/1 -> Logical Operator28/1

== matlab function PvtSubSys_VSM_ACC_DHT/Subsystem/ACC_Condotion/MATLAB Function ==
  data: DriveBrake input; VehicleStandstill input; ActiveConditionsFulfilled output; ActiveEnable input
function ActiveConditionsFulfilled = fcn(DriveBrake,VehicleStandstill,ActiveEnable)
%#codegen
if DriveBrake
    if VehicleStandstill && ActiveEnable
        ActiveConditionsFulfilled = 1;
    else
        ActiveConditionsFulfilled = 0;
    end
else  
    if ActiveEnable
        ActiveConditionsFulfilled = 1;
    else
        ActiveConditionsFulfilled = 0;
    end   
end

== stateflow chart PvtSubSys_VSM_ACC_DHT/Subsystem/ACCTJA_SM/TJA_ACC1 ==
  state ACC_Main [parallel]
    settings: executionOrder=1
    state P
      (history)
      state Off
        entry:
        ACCSts=ACC_Off;
      state Passive
        state Reject
          entry:
          ACCSts=ACC_Reject;
          DriveOffReq=0;
        state Standby
          entry:
          ACCSts=ACC_Standby;
          DriveOffReq=0;
        (default) -> Reject
        Standby -> Reject [order 1] : [ACCActCondF_b==0]//抑制
        Reject -> Standby : [ACCActCondF_b==1]//无抑制
      (default) -> Off
      Off -> Passive : [((ACC_ON==true)||...
          | (TJA_ON==true))&&...
          | (VehConfigACC==1)]
      Passive -> Off : [((ACC_ON==false)&&...
          | (TJA_ON==false))||...
          | (VehConfigACC==0)]
    state Error
      entry:
      ACCSts=ACC_Failure;
    state ACC_Control
      state Brake_Only
        entry:
        BrakeOnlyNum=0;
        ACCSts=ACC_BrakeOnly;
        DriveOffReq=0;
        during:
        BrakeOnlyNum=min(BrakeOnlyNum+1,600);
      state Active
        entry:ActiveNum=1;
        state StandActive
          entry:
          ACCSts=ACC_StandActive;
          StandActiveNum=0;
          DriveOffReq=0;
          during:
          StandActiveNum=min(StandActiveNum+1,20000);
        state StandWait
          entry:
          ACCSts=ACC_StandWait;
          StandWaitNum=0;
          during:
          StandWaitNum=min(StandWaitNum+1,20000);
          exit:
          StandWaitNum=0;
        state ActiveControl
          entry:
          ACCSts=ACC_ActiveControl;
          ActiveControlNum=1;
          during:
          ActiveControlNum=min(ActiveControlNum+1,600);
          DriveOffReq=(DriveOffCondF_b*VehicleStandstill) || (CDDactive*VehicleStandstill*DriveOffReq*(ActiveControlNum<=200));
        state Suspend
          entry:
          ACCSts=ACC_Override;
          AccOverrideNum=0;
          during:
          AccOverrideNum=min(45000,AccOverrideNum+1);
          DriveOffReq=CDDactive*VehicleStandstill*DriveOffReq*(ActiveControlNum<=200);
          exit:
          AccOverrideNum=0;
        StandActive -> Suspend [order 3] : [AccOverride==1]
        (junction 263) -> StandActive [order 2]
        ActiveControl -> StandActive [order 1] : [(VehicleStandstill==1)&&...
            | (DriverBrake==0)&&...
            | (DriveOffCondF_b~=1)]
        StandActive -> ActiveControl [order 1] : [(DriveOffCondF_b==1)&&...
            | (StandActive2Active_DrvrSts==1)&&...
            | (DriverBrake==0)]/DriveOffReq=1;
        StandActive -> StandWait [order 2] : [(VehicleStandstill==1)&&...
            | ((StandActiveNum>...
            | ACC_StandActiveNum)||...
            | (StandActive2Wait_Environ==1))]
        StandWait -> StandActive [order 1] : [(DriverBrake==0)&&...
            | (DriveOffCondF_b==0)&&...
            | ((AccPedalTouch==1)||(Switch_Res==true))]
        StandWait -> Suspend [order 2] : [AccOverride==1]
        StandWait -> ActiveControl [order 3] : [(DriverBrake==0)&&...
            | (DriveOffCondF_b==1)&&...
            | ((AccPedalTouch==1)||...
            | (Switch_Res==true))]...
            | /DriveOffReq=1;
        ActiveControl -> StandWait [order 3] : [(VehicleStandstill==1)&&...
            | (DriverBrake==1)]
        (default) -> (junction 261)
        (junction 261) -> (junction 263) [order 2]
        (junction 263) -> ActiveControl [order 1] : [VehicleStandstill==0]
        (junction 261) -> Suspend [order 1] : [AccOverride==1]
        Suspend -> ActiveControl [order 2] : [AccOverride==0]
        ActiveControl -> Suspend [order 4] : [AccOverride==1]
      ActiveControl -> Brake_Only [order 2] : [(ACCSlowExit_b==1)&&...
          | (ACCDecEnableBOM==1)]
    (default) -> P
    Error -> P : [ACCFailure==0]
    P -> Error : [ACCFailure==1]
    ACC_Control -> Off [order 2] : [(ACC_ON==false)&&...
        | (TJA_ON==false)]
    ACC_Control -> Error [order 1] : [TJAActive~=1&&...
        | ACCFailure==1]
    Suspend -> Passive [order 1] : [ACCSlowExit_b==1]
    Standby -> (junction 259) [order 2] : [(ACC_ON==true)&&...
        | (Switch_Set==true)]
    Standby -> (junction 259) [order 3] : [(ACC_ON==true)&&...
        | (Switch_Res==true)&&...//Res了
        | (ActiveNum>0)]//ActiveNum用以区分激活还是复位
    Brake_Only -> Passive : [(BrakeOnlyNum>P_VSM_ACC_BrakeOnlyNum)||...//breakonly超过10s
        | (ACCDecDisableBOM==1)||...
        | (AccOverride==1)||...
        | (VehicleStandstill==1)||...//车辆静止
        | (NoTarget==1)||...//无目标
        | (ACCFastExit_b==1)]
    Active -> Passive : [(ACCFastExit_b==1)||...
        | ((ACCSlowExit_b==1)&&...
        | (ACCDecEnableBOM~=1))]
    (junction 259) -> Active
  data: StandActiveNum local uint16; ACC_ON input boolean size=1; TJA_ON input boolean size=1; CDDactive input size=1; VehicleStandstill input size=1; ACCFailure input size=1; ACCActCondF_b input size=1; DriveOffCondF_b input size=1; AccOverride input size=1; ActiveNum local uint16 size=1 [0..100] =0; ACCFastExit_b input size=1; ACCSlowExit_b input size=1; StandWaitNum output uint16 size=1 =0; ActiveControlNum local uint16 size=1 =0; BrakeOnlyNum local uint16 size=1 =0; DriverBrake input size=1; DriveOffReq output boolean size=1 =0; NoTarget input size=1; AccPedalTouch input size=1; ACCSts output Enum: ACC_STATE size=1 =ACC_STATE.ACC_Off; Switch_Set input boolean size=1 =false; Switch_Res input boolean size=1 =false; VehConfigTJA input boolean; VehConfigACC input boolean; ACCDecEnableBOM input boolean size=1; ACCDecDisableBOM input boolean size=1; ActiveWaitNum local uint16 size=1; AccOverrideNum local uint16 size=1 [0..100] =0; P_VSM_ACC_BrakeOnlyNum parameter uint16; ACC_StandActiveNum input; StandActive2Wait_Environ input; StandActive2Active_DrvrSts input; cnt local uint16; SafeStopNum local uint16; TJAActive input boolean

== stateflow chart PvtSubSys_VSM_ACC_DHT/Subsystem/ACCTJA_SM/TJA_ACC2 ==
  state TJA_Main [parallel]
    settings: executionOrder=1
    state Off
      en:
      TJASts=TJA_Off;
    state TJAOn
      state Error
        en:
        TJASts=TJA_Error;
      state W
        state Ready
          en:
          TJASts=TJA_Ready;
        state Idle
          en:
          TJASts=TJA_Idle;
        state Active
          en:
          TJASts=TJA_Active;
          cnt=0;
          du:
          cnt=min(10,cnt+1)
        state Wait
          en:
          TJASts=TJA_Wait;
          du:
          ActiveWaitNum=min(3000,ActiveWaitNum+1);
          ex:
          ActiveWaitNum=0;
        state Idle1
          en:
          TJASts=TJA_Idle;
          TJASafeStopExit_b=false;
        state Recover
          en:
          TJASts=TJA_Ready;
        state SafeStop
          en:
          TJASts=TJA_SafeStop;
          du:
          SafeStopNum=min(300,SafeStopNum+1);
          TJASafeStopExit_b=(SafeStopNum>250);
          ACCParkShiftReq_b=VehicleStandstill;
          ex:
          TJAStopExit=true;
          ACCParkShiftReq_b=false;
          SafeStopNum=0;
        (junction 438) -> Idle [order 1] : [(ACCSts==ACC_Reject)||...
            | (TJA_LCKState~=LCK_STATE.LCK_Active)||...
            | (TJASafeStopExit_b==true)||...
            | (ESSState==4||ESSState==5)]
        (junction 438) -> Ready [order 2] : [(ACCSts~=ACC_Reject)&&...
            | (TJA_LCKState==LCK_STATE.LCK_Active)&&...
            | (TJASafeStopExit_b==false)]
        Ready -> Idle [order 2] : [(ACCSts==ACC_Reject)||...
            | (TJA_LCKState~=LCK_STATE.LCK_Active)]
        Ready -> TJA_Main.TJAOn.W.Active [order 1] : [Switch_SetTJA==true]
        Idle -> Ready [order 2] : [(ACCSts~=ACC_Reject)&&...
            | (TJA_LCKState==LCK_STATE.LCK_Active)&&...
            | (TJASafeStopExit_b==false)&&...
            | (ESSState~=4&&ESSState~=5)]
        Wait -> Ready [order 2] : [(ActiveWaitNum>=...
            | P_VSM_TJA_ActiveWaitNum)||...
            | (ACCSts==ACC_Standby)]
        TJA_Main.TJAOn.W.Active -> Wait [order 5] : [LCKSts~=LCK_Active&&...
            | cnt>2]
        Wait -> TJA_Main.TJAOn.W.Active [order 4] : [LCKSts==LCK_Active]
        Wait -> Idle [order 1] : [ACCSts==ACC_Reject]
        TJA_Main.TJAOn.W.Active -> Ready [order 3] : [(ACCSts==ACC_Standby)]
        Recover -> Ready [order 3] : [(ACCSts==ACC_Standby)]
        Recover -> Wait [order 1] : [ACCSts==ACC_ActiveControl]
        Wait -> Recover [order 3] : [(ACCSts==ACC_StandWait)]
        Idle -> Idle1 [order 1] : [TJASafeStopExit_b==true&&...
            | Gear_P==true]
        Idle1 -> Idle : [Gear_P==false]
        Recover -> Idle [order 2] : [(ACCSts==ACC_Reject)]
        TJA_Main.TJAOn.W.Active -> Recover [order 4] : [ACCSts==ACC_StandWait]
        SafeStop -> Idle : [(HandsOff_b==0)||...
            | (StandWaitNum>1500)||...
            | (ACCSts==ACC_Reject)||...
            | (AccOverrideNum>3000)]
        TJA_Main.TJAOn.W.Active -> SafeStop [order 2] : [HandsOffWarnLevel==4]
        (junction 523) -> Idle [order 2] : [HWAStopExit==true]
        TJA_Main.TJAOn.W.Active -> (junction 523) [order 1]
        (junction 523) -> Idle [order 1] : [(ACCSts==ACC_Reject)||...
            | (ESSState==4||ESSState==5)]
      TJA_Main.TJAOn.Error -> (junction 521) : [(ACCSts!=ACC_Failure)&&(LCKSts!=LCK_Error)]
      (junction 521) -> (junction 464)
      (junction 464) -> TJA_Main.TJAOn.Error [order 1] : [(ACCSts==ACC_Failure)||(LCKSts==LCK_Error)]
      (junction 464) -> (junction 438) [order 2]
      W -> TJA_Main.TJAOn.Error : [(ACCSts==ACC_Failure)||...
          | (LCKSts==LCK_Error)]
    (default) -> TJA_Main.Off
    TJAOn -> TJA_Main.Off : [(TJA_ON==false)||(VehConfigTJA==0)]
    TJA_Main.Off -> (junction 521) : [(TJA_ON==true)&&(VehConfigTJA==1)]
  state ACC_Main [parallel]
    settings: executionOrder=2
    state P
      (history)
      state Off
        entry:
        ACCSts=ACC_Off;
      state Passive
        state Reject
          entry:
          ACCSts=ACC_Reject;
          TJAStopExit=false;
          DriveOffReq=0;
        state Standby
          entry:
          ACCSts=ACC_Standby;
          TJAStopExit=false;
          DriveOffReq=0;
        (default) -> Reject
        Standby -> Reject [order 1] : [ACCActCondF_b==0]//抑制
        Reject -> Standby : [ACCActCondF_b==1]//无抑制
      (default) -> ACC_Main.P.Off
      ACC_Main.P.Off -> Passive : [((ACC_ON==true)||...
          | (TJA_ON==true))&&...
          | (VehConfigACC==1)]
      Passive -> ACC_Main.P.Off : [((ACC_ON==false)&&...
          | (TJA_ON==false))||...
          | (VehConfigACC==0)]
    state Error
      entry:
      ACCSts=ACC_Failure;
    state ACC_Control
      state Brake_Only
        entry:
        BrakeOnlyNum=0;
        ACCSts=ACC_BrakeOnly;
        DriveOffReq=0;
        during:
        BrakeOnlyNum=min(BrakeOnlyNum+1,600);
      state Active
        entry:ActiveNum=1;
        state StandActive
          entry:
          ACCSts=ACC_StandActive;
          StandActiveNum=0;
          DriveOffReq=0;
          during:
          StandActiveNum=min(StandActiveNum+1,20000);
        state StandWait
          entry:
          ACCSts=ACC_StandWait;
          StandWaitNum=0;
          during:
          StandWaitNum=min(StandWaitNum+1,20000);
          exit:
          StandWaitNum=0;
        state ActiveControl
          entry:
          ACCSts=ACC_ActiveControl;
          ActiveControlNum=1;
          during:
          ActiveControlNum=min(ActiveControlNum+1,600);
          DriveOffReq=(DriveOffCondF_b*VehicleStandstill) || (CDDactive*VehicleStandstill*DriveOffReq*(ActiveControlNum<=200));
        state Suspend
          entry:
          ACCSts=ACC_Override;
          AccOverrideNum=0;
          during:
          AccOverrideNum=min(45000,AccOverrideNum+1);
          DriveOffReq=CDDactive*VehicleStandstill*DriveOffReq*(ActiveControlNum<=200);
          exit:
          AccOverrideNum=0;
        StandActive -> Suspend [order 3] : [AccOverride==1]
        (junction 263) -> StandActive [order 2]
        ActiveControl -> StandActive [order 1] : [(VehicleStandstill==1)&&...
            | (DriverBrake==0)&&...
            | (DriveOffCondF_b~=1)]
        StandActive -> ActiveControl [order 1] : [(DriveOffCondF_b==1)&&...
            | (StandActive2Active_DrvrSts==1)&&...
            | (DriverBrake==0)]/DriveOffReq=1;
        StandActive -> StandWait [order 2] : [(VehicleStandstill==1)&&...
            | ((StandActiveNum>...
            | ACC_StandActiveNum)||...
            | (StandActive2Wait_Environ==1))]
        StandWait -> StandActive [order 1] : [(DriverBrake==0)&&...
            | (DriveOffCondF_b==0)&&...
            | ((AccPedalTouch==1)||(Switch_Res==true))]
        StandWait -> Suspend [order 2] : [AccOverride==1]
        StandWait -> ActiveControl [order 3] : [(DriverBrake==0)&&...
            | (DriveOffCondF_b==1)&&...
            | ((AccPedalTouch==1)||...
            | (Switch_Res==true))]...
            | /DriveOffReq=1;
        ActiveControl -> StandWait [order 3] : [(VehicleStandstill==1)&&...
            | (DriverBrake==1)]
        (default) -> (junction 261)
        (junction 261) -> (junction 263) [order 2]
        (junction 263) -> ActiveControl [order 1] : [VehicleStandstill==0]
        (junction 261) -> Suspend [order 1] : [AccOverride==1]
        Suspend -> ActiveControl [order 2] : [AccOverride==0]
        ActiveControl -> Suspend [order 4] : [AccOverride==1]
      ActiveControl -> Brake_Only [order 2] : [(ACCSlowExit_b==1)&&...
          | (ACCDecEnableBOM==1)]
    (default) -> P
    ACC_Main.Error -> P : [ACCFailure==0]
    P -> ACC_Main.Error : [ACCFailure==1]
    ACC_Control -> ACC_Main.P.Off [order 2] : [(ACC_ON==false)&&...
        | (TJA_ON==false)]
    ACC_Control -> ACC_Main.Error [order 1] : [HWAActive~=1&&...
        | ACCFailure==1]
    Suspend -> Passive [order 1] : [ACCSlowExit_b==1]
    Standby -> (junction 259) [order 2] : [(ACC_ON==true)&&...
        | (Switch_Set==true)]
    Standby -> (junction 259) [order 3] : [(ACC_ON==true)&&...
        | (Switch_Res==true)&&...//Res了
        | (ActiveNum>0)]//ActiveNum用以区分激活还是复位
    ACC_Control -> Reject [commented out] : [(HWAStopExit==true)||...//HWA的调度
        | (TJAStopExit==true)]//TJA的调度
    Brake_Only -> Passive : [(BrakeOnlyNum>P_VSM_ACC_BrakeOnlyNum)||...//breakonly超过10s
        | (ACCDecDisableBOM==1)||...
        | (AccOverride==1)||...
        | (VehicleStandstill==1)||...//车辆静止
        | (NoTarget==1)||...//无目标
        | (ACCFastExit_b==1)]
    ACC_Main.ACC_Control.Active -> Passive : [(ACCFastExit_b==1)||...
        | ((ACCSlowExit_b==1)&&...
        | (ACCDecEnableBOM~=1))]
    (junction 259) -> ACC_Main.ACC_Control.Active
  data: StandActiveNum local uint16; ACC_ON input boolean size=1; TJA_ON input boolean size=1; CDDactive input size=1; VehicleStandstill input size=1; ACCFailure input size=1; ACCActCondF_b input size=1; DriveOffCondF_b input size=1; AccOverride input size=1; ActiveNum local uint16 size=1 [0..100] =0; ACCFastExit_b input size=1; ACCSlowExit_b input size=1; StandWaitNum output uint16 size=1 =0; ActiveControlNum local uint16 size=1 =0; BrakeOnlyNum local uint16 size=1 =0; DriverBrake input size=1; DriveOffReq output boolean size=1 =0; NoTarget input size=1; AccPedalTouch input size=1; ACCSts output Enum: ACC_STATE size=1 =ACC_STATE.ACC_Off; TJASts output Enum: TJA_STATE size=1 =TJA_STATE.TJA_Off; TJASafeStopExit_b output boolean size=1 =false; LCKSts input Enum: LCK_STATE size=1; HandsOffWarnLevel input uint8 size=1; TJAStopExit local boolean size=1 =false; Switch_Set input boolean size=1 =false; Switch_Res input boolean size=1 =false; HWAStopExit input boolean size=1 =false; ACCParkShiftReq_b output boolean size=1 =0; HWAActive input boolean size=1 =false; HandsOff_b input boolean size=1 =false; HWADriveOffCondF_b input boolean size=1 =false; VehConfigTJA input boolean; VehConfigACC input boolean; ACCDecEnableBOM input boolean size=1; ACCDecDisableBOM input boolean size=1; Switch_SetTJA input boolean; Gear_P input; ActiveWaitNum local uint16 size=1; ESSState input; TJA_LCKState input; AccOverrideNum local uint16 size=1 [0..100] =0; P_VSM_ACC_BrakeOnlyNum parameter uint16; P_VSM_TJA_ActiveWaitNum parameter uint16; ACC_StandActiveNum input; StandActive2Wait_Environ input; StandActive2Active_DrvrSts input; cnt local uint16; SafeStopNum local uint16
